simulink model "Drone2_simulink_old1"  (R2024b)
settings: Solver=ode1be  StartTime=0.0  StopTime=1200  FixedStep=0.001  MaxStep=0.001  MinStep=0.00095  RelTol=1e-3
undefined symbols (not defined in the file): DiscIntNeverNeededParam, Environment, Newton, Raphson, Sim3dSensor, Vehicle, X, Y, Z
libraries: sm_lib x2951, nesl_utility x76, slpidlib x25, simulink x4, eeGeneralControl x4, matrix_library x3, rllib x2, sim3dlib x2, uavsim3dlib x2, dspstat3 x1, SignalEditorBlockLib x1, sharedutil x1
(part 9 of 21)

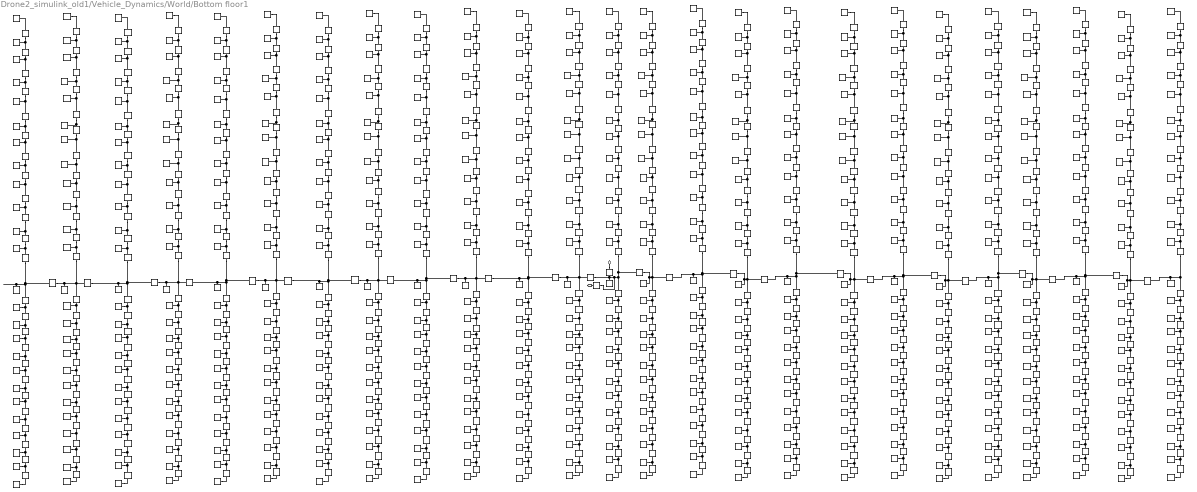
== system Drone2_simulink_old1/Vehicle_Dynamics/World/Bottom floor1 ==
  Brick Solid : sm_lib/Body Elements/Brick Solid  BrickDimensions=[25*X 25*Y Z]  BrickDimensionsUnits=m  ExportEntireGeometry=on  InertiaType=CalculateFromGeometry  BasedOnType=Density  Density=10000  DensityUnits=kg/m^3  Mass=1  MassUnits=kg  CenterOfMass=[0 0 0]  CenterOfMassUnits=m  MomentsOfInertia=[1 1 1]  MomentsOfInertiaUnits=kg*m^2  ProductsOfInertia=[0 0 0]  ProductsOfInertiaUnits=kg*m^2  GraphicType=FromGeometry  MarkerShape=Sphere  MarkerSize=10  GraphicVisPropType=SimpleVisualProperties  GraphicDiffuseColor=[1.0 1.0 1.0]  GraphicOpacity=0  GraphicSpecularColor=[0.5 0.5 0.5 1.0]  GraphicAmbientColor=[0.15 0.15 0.15 1.0]  GraphicEmissiveColor=[0.0 0.0 0.0 1.0]  GraphicShininess=75  DoExposeReferenceFrame=on  SerializedFrames=<Frames/>
  Rigid Transform : sm_lib/Frames and Transforms/Rigid Transform  RotationMethod=None  FollAlignAxisA=+X  BaseAlignAxisA=+Y  FollAlignAxisB=+Y  BaseAlignAxisB=+Z  RotationStandardAxis=+Z  RotationAngle=0  RotationAngleUnits=deg  RotationArbitraryAxis=[0 0 1]  RotationSequenceAxes=FollowerAxes  RotationSequence=XYX  RotationSequenceAngles=[0 0 0]  RotationSequenceAnglesUnits=deg  RotationMatrix=[1 0 0;0 1 0;0 0 1]  Quaternion=[1 0 0 0]  TranslationMethod=Cartesian  TranslationCartesianOffset=[0 0 ZB]  TranslationCartesianOffsetUnits=m  TranslationStandardAxis=+Z  TranslationStandardOffset=0  TranslationStandardOffsetUnits=m  TranslationROffset=0  TranslationROffsetUnits=m  TranslationThetaOffset=0  TranslationThetaOffsetUnits=deg  TranslationZOffset=0  TranslationZOffsetUnits=m
  Rigid Transform{1,5,7,9..10,12..13,15..16,18..19,21} (12 alike) : sm_lib/Frames and Transforms/Rigid Transform  RotationMethod=None  FollAlignAxisA=+X  BaseAlignAxisA=+Y  FollAlignAxisB=+Y  BaseAlignAxisB=+Z  RotationStandardAxis=+Z  RotationAngle=0  RotationAngleUnits=deg  RotationArbitraryAxis=[0 0 1]  RotationSequenceAxes=FollowerAxes  RotationSequence=XYX  RotationSequenceAngles=[0 0 0]  RotationSequenceAnglesUnits=deg  RotationMatrix=[1 0 0;0 1 0;0 0 1]  Quaternion=[1 0 0 0]  TranslationMethod=Cartesian  TranslationCartesianOffset=[X 0 0]  TranslationCartesianOffsetUnits=m  TranslationStandardAxis=+Z  TranslationStandardOffset=0  TranslationStandardOffsetUnits=m  TranslationROffset=0  TranslationROffsetUnits=m  TranslationThetaOffset=0  TranslationThetaOffsetUnits=deg  TranslationZOffset=0  TranslationZOffsetUnits=m
  Rigid Transform{2..4,6,8,11,14,17,20,22..24} (12 alike) : sm_lib/Frames and Transforms/Rigid Transform  RotationMethod=None  FollAlignAxisA=+X  BaseAlignAxisA=+Y  FollAlignAxisB=+Y  BaseAlignAxisB=+Z  RotationStandardAxis=+Z  RotationAngle=0  RotationAngleUnits=deg  RotationArbitraryAxis=[0 0 1]  RotationSequenceAxes=FollowerAxes  RotationSequence=XYX  RotationSequenceAngles=[0 0 0]  RotationSequenceAnglesUnits=deg  RotationMatrix=[1 0 0;0 1 0;0 0 1]  Quaternion=[1 0 0 0]  TranslationMethod=Cartesian  TranslationCartesianOffset=[-X 0 0]  TranslationCartesianOffsetUnits=m  TranslationStandardAxis=+Z  TranslationStandardOffset=0  TranslationStandardOffsetUnits=m  TranslationROffset=0  TranslationROffsetUnits=m  TranslationThetaOffset=0  TranslationThetaOffsetUnits=deg  TranslationZOffset=0  TranslationZOffsetUnits=m
  bottom{,3..4,6,8,10,13,15,17,19,21,23..25,27,30,32,34,36,41..44,46,48,50,52,55,57,59,61,66..69,71,73,75,77,80,82,84,86,89,91..94,96,98,100,102,105,107,109,111,114,116..119,121,123,125,127,130,132,134,136,141..144,146,148,150,152,155,157,159,161,164,166..169,171,173,175,177,180,182,184,186,191..194,196,198,200,202,205,207,209,211,214,216..219,221,223,225,227,230,232,234,236,241..244,246,248,250,252,255,257,259,261,264,266..269,271,273,275,277,280,282,284,286,291..294,296,298,300,302,305,307,309,311,314,316..319,321,323,325,327,330,332,334,336,341..344,346,348,350,352,355,357,359,361,364,366..369,371,373,375,377,380,382,384,386,389,391..394,396,398,400,402,405,407,409,411,416..419,421,423,425,427,430,432,434,436,439,441..444,446,448,450,452,455,457,459,461,464,466..469,471,473,475,477,480,482,484,486,491..494,496,498,500,502,505,507,509,511,516..519,521,523,525,527,530,532,534,536,539,541..544,546,548,550,552,555,557,559,561,564,566..569,571,573,575,577,580,582,584,586,591..594,596,598,600,602,605,607,609,611,616..619,621,623} (313 alike) : sm_lib/Body Elements/Brick Solid  BrickDimensions=[X Y Z]  BrickDimensionsUnits=m  ExportEntireGeometry=off  InertiaType=CalculateFromGeometry  BasedOnType=Density  Density=1  DensityUnits=kg/m^3  Mass=1  MassUnits=kg  CenterOfMass=[0 0 0]  CenterOfMassUnits=m  MomentsOfInertia=[1 1 1]  MomentsOfInertiaUnits=kg*m^2  ProductsOfInertia=[0 0 0]  ProductsOfInertiaUnits=kg*m^2  GraphicType=FromGeometry  MarkerShape=Sphere  MarkerSize=10  GraphicVisPropType=SimpleVisualProperties  GraphicDiffuseColor=Color1  GraphicOpacity=1  GraphicSpecularColor=[0.5 0.5 0.5 1.0]  GraphicAmbientColor=[0.15 0.15 0.15 1.0]  GraphicEmissiveColor=[0.0 0.0 0.0 1.0]  GraphicShininess=75  DoExposeReferenceFrame=on  SerializedFrames=<Frames/>
  bottom{1..2,5,7,9,11..12,14,16,18,20,22,26,28..29,31,33,35,37..40,45,47,49,51,53..54,56,58,60,62..65,70,72,74,76,78..79,81,83,85,87..88,90,95,97,99,101,103..104,106,108,110,112..113,115,120,122,124,126,128..129,131,133,135,137..140,145,147,149,151,153..154,156,158,160,162..163,165,170,172,174,176,178..179,181,183,185,187..190,195,197,199,201,203..204,206,208,210,212..213,215,220,222,224,226,228..229,231,233,235,237..240,245,247,249,251,253..254,256,258,260,262..263,265,270,272,274,276,278..279,281,283,285,287..290,295,297,299,301,303..304,306,308,310,312..313,315,320,322,324,326,328..329,331,333,335,337..340,345,347,349,351,353..354,356,358,360,362..363,365,370,372,374,376,378..379,381,383,385,387..388,390,395,397,399,401,403..404,406,408,410,412..415,420,422,424,426,428..429,431,433,435,437..438,440,445,447,449,451,453..454,456,458,460,462..463,465,470,472,474,476,478..479,481,483,485,487..490,495,497,499,501,503..504,506,508,510,512..515,520,522,524,526,528..529,531,533,535,537..538,540,545,547,549,551,553..554,556,558,560,562..563,565,570,572,574,576,578..579,581,583,585,587..590,595,597,599,601,603..604,606,608,610,612..615,620,622,624} (312 alike) : sm_lib/Body Elements/Brick Solid  BrickDimensions=[X Y Z]  BrickDimensionsUnits=m  ExportEntireGeometry=off  InertiaType=CalculateFromGeometry  BasedOnType=Density  Density=1  DensityUnits=kg/m^3  Mass=1  MassUnits=kg  CenterOfMass=[0 0 0]  CenterOfMassUnits=m  MomentsOfInertia=[1 1 1]  MomentsOfInertiaUnits=kg*m^2  ProductsOfInertia=[0 0 0]  ProductsOfInertiaUnits=kg*m^2  GraphicType=FromGeometry  MarkerShape=Sphere  MarkerSize=10  GraphicVisPropType=SimpleVisualProperties  GraphicDiffuseColor=Color2  GraphicOpacity=1  GraphicSpecularColor=[0.5 0.5 0.5 1.0]  GraphicAmbientColor=[0.15 0.15 0.15 1.0]  GraphicEmissiveColor=[0.0 0.0 0.0 1.0]  GraphicShininess=75  DoExposeReferenceFrame=on  SerializedFrames=<Frames/>
  water surface ti bottom{1..2,4..5,7..10,12..13,18,24,26,28..29,34,36..37,41,43..44,46..48,50,52..53,58,60..61,65,67..68,70..74,76..77,82,84,89,91..92,94..98,100..101,106,108,113,115..116,118..120,122,124..125,130,132..133,137,139..140,142..146,148..149,154,156,161,163..164,166..168,170,172..173,178,180..181,185,187..188,190..194,196..197,202,204,209,211..212,214..216,218,220..221,226,228..229,233,235..236,238..242,244..245,250,252,257,259..260,262..264,266,268..269,274,276..277,281,283..284,286..290,292..293,298,300,305,307..308,310..312,314,316..317,322,324..325,329,331..332,334..338,340..341,346,348,353,355..356,358..362,367,369,374,376..377,379..381,383,385..386,391,393..394,398,400..401,403..407,409..410,415,417,422,424..425,427..431,436,438,443,445..446,448..450,452,454..455,460,462..463,467,469..470,472..476,479,481..482,487,489..490,494,496..497,499..503,505..506,511,513,518,520..521,523..527,532,534,539,541..542,544..546,548,550..551,556,558..559,563,565..566,568..572,575,577..578,583,585..586,590,592..593,595..599} (300 alike) : sm_lib/Frames and Transforms/Rigid Transform  RotationMethod=None  FollAlignAxisA=+X  BaseAlignAxisA=+Y  FollAlignAxisB=+Y  BaseAlignAxisB=+Z  RotationStandardAxis=+Z  RotationAngle=0  RotationAngleUnits=deg  RotationArbitraryAxis=[0 0 1]  RotationSequenceAxes=FollowerAxes  RotationSequence=XYX  RotationSequenceAngles=[0 0 0]  RotationSequenceAnglesUnits=deg  RotationMatrix=[1 0 0;0 1 0;0 0 1]  Quaternion=[1 0 0 0]  TranslationMethod=Cartesian  TranslationCartesianOffset=[0 Y 0]  TranslationCartesianOffsetUnits=m  TranslationStandardAxis=+Z  TranslationStandardOffset=0  TranslationStandardOffsetUnits=m  TranslationROffset=0  TranslationROffsetUnits=m  TranslationThetaOffset=0  TranslationThetaOffsetUnits=deg  TranslationZOffset=0  TranslationZOffsetUnits=m
  water surface ti bottom{3,6,11,14..17,19..23,25,27,30..33,35,38..40,42,45,49,51,54..57,59,62..64,66,69,75,78..81,83,85..88,90,93,99,102..105,107,109..112,114,117,121,123,126..129,131,134..136,138,141,147,150..153,155,157..160,162,165,169,171,174..177,179,182..184,186,189,195,198..201,203,205..208,210,213,217,219,222..225,227,230..232,234,237,243,246..249,251,253..256,258,261,265,267,270..273,275,278..280,282,285,291,294..297,299,301..304,306,309,313,315,318..321,323,326..328,330,333,339,342..345,347,349..352,354,357,363..366,368,370..373,375,378,382,384,387..390,392,395..397,399,402,408,411..414,416,418..421,423,426,432..435,437,439..442,444,447,451,453,456..459,461,464..466,468,471,477..478,480,483..486,488,491..493,495,498,504,507..510,512,514..517,519,522,528..531,533,535..538,540,543,547,549,552..555,557,560..562,564,567,573..574,576,579..582,584,587..589,591,594,600} (300 alike) : sm_lib/Frames and Transforms/Rigid Transform  RotationMethod=None  FollAlignAxisA=+X  BaseAlignAxisA=+Y  FollAlignAxisB=+Y  BaseAlignAxisB=+Z  RotationStandardAxis=+Z  RotationAngle=0  RotationAngleUnits=deg  RotationArbitraryAxis=[0 0 1]  RotationSequenceAxes=FollowerAxes  RotationSequence=XYX  RotationSequenceAngles=[0 0 0]  RotationSequenceAnglesUnits=deg  RotationMatrix=[1 0 0;0 1 0;0 0 1]  Quaternion=[1 0 0 0]  TranslationMethod=Cartesian  TranslationCartesianOffset=[0 -Y 0]  TranslationCartesianOffsetUnits=m  TranslationStandardAxis=+Z  TranslationStandardOffset=0  TranslationStandardOffsetUnits=m  TranslationROffset=0  TranslationROffsetUnits=m  TranslationThetaOffset=0  TranslationThetaOffsetUnits=deg  TranslationZOffset=0  TranslationZOffsetUnits=m
  From World : PMIOPort  Side=Left
  Collision : PMIOPort  Port=2  Side=Right
  connections:
  Collision/RConn1 -- Brick Solid/LConn1
  bottom539/RConn1 -- water surface ti bottom514/RConn1
  water surface ti bottom539/RConn1 -- bottom567/RConn1
  water surface ti bottom518/RConn1 -- bottom542/RConn1
  bottom589/RConn1 -- water surface ti bottom559/RConn1
  bottom588/RConn1 -- water surface ti bottom560/RConn1
  bottom564/RConn1 -- water surface ti bottom535/RConn1
  bottom613/RConn1 -- water surface ti bottom587/RConn1
  bottom614/RConn1 -- water surface ti bottom586/RConn1
  water surface ti bottom535/LConn1 -- water surface ti bottom536/RConn1 -- bottom563/RConn1
  water surface ti bottom536/LConn1 -- bottom566/RConn1 -- water surface ti bottom537/RConn1
  water surface ti bottom537/LConn1 -- bottom565/RConn1 -- water surface ti bottom538/RConn1
  water surface ti bottom529/RConn1 -- bottom559/RConn1 -- water surface ti bottom538/LConn1
  water surface ti bottom529/LConn1 -- bottom558/RConn1 -- water surface ti bottom530/RConn1
  water surface ti bottom530/LConn1 -- water surface ti bottom531/RConn1 -- bottom561/RConn1
  water surface ti bottom531/LConn1 -- water surface ti bottom533/RConn1 -- bottom560/RConn1
  water surface ti bottom533/LConn1 -- bottom557/RConn1 -- water surface ti bottom573/RConn1
  water surface ti bottom573/LConn1 -- water surface ti bottom528/RConn1 -- bottom554/RConn1
  water surface ti bottom539/LConn1 -- bottom556/RConn1 -- water surface ti bottom527/RConn1
  water surface ti bottom527/LConn1 -- water surface ti bottom526/RConn1 -- bottom555/RConn1
  bottom553/RConn1 -- water surface ti bottom526/LConn1 -- water surface ti bottom532/RConn1
  water surface ti bottom532/LConn1 -- bottom552/RConn1 -- water surface ti bottom572/RConn1
  water surface ti bottom546/RConn1 -- bottom574/RConn1 -- water surface ti bottom572/LConn1
  water surface ti bottom545/RConn1 -- bottom573/RConn1 -- water surface ti bottom546/LConn1
  water surface ti bottom545/LConn1 -- water surface ti bottom544/RConn1 -- bottom572/RConn1
  water surface ti bottom542/RConn1 -- bottom571/RConn1 -- water surface ti bottom544/LConn1
  water surface ti bottom542/LConn1 -- water surface ti bottom541/RConn1 -- bottom570/RConn1
  water surface ti bottom528/LConn1 -- bottom569/RConn1 -- water surface ti bottom540/RConn1
  water surface ti bottom534/RConn1 -- bottom568/RConn1 -- water surface ti bottom541/LConn1
  bottom550/RConn1 -- water surface ti bottom543/LConn1 -- water surface ti bottom571/LConn1 -- Rigid Transform23/RConn1
  water surface ti bottom571/RConn1 -- bottom551/RConn1 -- water surface ti bottom534/LConn1
  water surface ti bottom540/LConn1 -- bottom562/RConn1 -- water surface ti bottom543/RConn1
  water surface ti bottom559/LConn1 -- water surface ti bottom563/RConn1 -- bottom592/RConn1
  water surface ti bottom560/LConn1 -- bottom591/RConn1 -- water surface ti bottom561/RConn1
  water surface ti bottom561/LConn1 -- bottom590/RConn1 -- water surface ti bottom562/RConn1
  water surface ti bottom553/RConn1 -- bottom584/RConn1 -- water surface ti bottom562/LConn1
  water surface ti bottom553/LConn1 -- bottom583/RConn1 -- water surface ti bottom554/RConn1
  water surface ti bottom554/LConn1 -- water surface ti bottom555/RConn1 -- bottom586/RConn1
  water surface ti bottom555/LConn1 -- water surface ti bottom557/RConn1 -- bottom585/RConn1
  water surface ti bottom557/LConn1 -- bottom582/RConn1 -- water surface ti bottom549/RConn1
  water surface ti bottom549/LConn1 -- water surface ti bottom552/RConn1 -- bottom579/RConn1
  water surface ti bottom551/RConn1 -- water surface ti bottom563/LConn1 -- bottom581/RConn1
  water surface ti bottom550/RConn1 -- water surface ti bottom551/LConn1 -- bottom580/RConn1
  water surface ti bottom556/RConn1 -- water surface ti bottom550/LConn1 -- bottom578/RConn1
  water surface ti bottom548/RConn1 -- water surface ti bottom556/LConn1 -- bottom577/RConn1
  water surface ti bottom548/LConn1 -- water surface ti bottom570/RConn1 -- bottom599/RConn1
  water surface ti bottom570/LConn1 -- water surface ti bottom569/RConn1 -- bottom598/RConn1
  water surface ti bottom568/RConn1 -- water surface ti bottom569/LConn1 -- bottom597/RConn1
  water surface ti bottom566/RConn1 -- water surface ti bottom568/LConn1 -- bottom596/RConn1
  water surface ti bottom565/RConn1 -- water surface ti bottom566/LConn1 -- bottom595/RConn1
  water surface ti bottom552/LConn1 -- bottom594/RConn1 -- water surface ti bottom564/RConn1
  water surface ti bottom558/RConn1 -- water surface ti bottom565/LConn1 -- bottom593/RConn1
  water surface ti bottom567/LConn1 -- water surface ti bottom547/RConn1 -- bottom575/RConn1
  Rigid Transform20/RConn1 -- water surface ti bottom558/LConn1 -- Rigid Transform23/LConn1 -- bottom576/RConn1 -- water surface ti bottom547/LConn1
  bottom587/RConn1 -- water surface ti bottom564/LConn1 -- water surface ti bottom567/RConn1
  water surface ti bottom514/LConn1 -- bottom538/RConn1 -- water surface ti bottom515/RConn1
  water surface ti bottom515/LConn1 -- water surface ti bottom516/RConn1 -- bottom541/RConn1
  water surface ti bottom516/LConn1 -- water surface ti bottom517/RConn1 -- bottom540/RConn1
  water surface ti bottom508/RConn1 -- water surface ti bottom517/LConn1 -- bottom534/RConn1
  water surface ti bottom508/LConn1 -- water surface ti bottom509/RConn1 -- bottom533/RConn1
  water surface ti bottom509/LConn1 -- bottom536/RConn1 -- water surface ti bottom510/RConn1
  water surface ti bottom510/LConn1 -- bottom535/RConn1 -- water surface ti bottom512/RConn1
  water surface ti bottom512/LConn1 -- water surface ti bottom600/RConn1 -- bottom532/RConn1
  water surface ti bottom600/LConn1 -- bottom529/RConn1 -- water surface ti bottom507/RConn1
  water surface ti bottom518/LConn1 -- water surface ti bottom506/RConn1 -- bottom531/RConn1
  water surface ti bottom506/LConn1 -- bottom530/RConn1 -- water surface ti bottom505/RConn1
  bottom528/RConn1 -- water surface ti bottom511/RConn1 -- water surface ti bottom505/LConn1
  water surface ti bottom511/LConn1 -- water surface ti bottom599/RConn1 -- bottom527/RConn1
  water surface ti bottom525/RConn1 -- water surface ti bottom599/LConn1 -- bottom549/RConn1
  water surface ti bottom524/RConn1 -- water surface ti bottom525/LConn1 -- bottom548/RConn1
  water surface ti bottom524/LConn1 -- bottom547/RConn1 -- water surface ti bottom523/RConn1
  water surface ti bottom521/RConn1 -- water surface ti bottom523/LConn1 -- bottom546/RConn1
  water surface ti bottom521/LConn1 -- bottom545/RConn1 -- water surface ti bottom520/RConn1
  water surface ti bottom507/LConn1 -- water surface ti bottom519/RConn1 -- bottom544/RConn1
  water surface ti bottom513/RConn1 -- water surface ti bottom520/LConn1 -- bottom543/RConn1
  water surface ti bottom598/LConn1 -- water surface ti bottom522/LConn1 -- bottom525/RConn1 -- Rigid Transform20/LConn1 -- Rigid Transform14/RConn1
  water surface ti bottom598/RConn1 -- water surface ti bottom513/LConn1 -- bottom526/RConn1
  water surface ti bottom519/LConn1 -- water surface ti bottom522/RConn1 -- bottom537/RConn1
  water surface ti bottom586/LConn1 -- bottom617/RConn1 -- water surface ti bottom590/RConn1
  water surface ti bottom587/LConn1 -- water surface ti bottom588/RConn1 -- bottom616/RConn1
  water surface ti bottom588/LConn1 -- water surface ti bottom589/RConn1 -- bottom615/RConn1
  water surface ti bottom580/RConn1 -- water surface ti bottom589/LConn1 -- bottom609/RConn1
  water surface ti bottom580/LConn1 -- water surface ti bottom581/RConn1 -- bottom608/RConn1
  water surface ti bottom581/LConn1 -- bottom611/RConn1 -- water surface ti bottom582/RConn1
  water surface ti bottom582/LConn1 -- bottom610/RConn1 -- water surface ti bottom584/RConn1
  water surface ti bottom584/LConn1 -- water surface ti bottom576/RConn1 -- bottom607/RConn1
  water surface ti bottom576/LConn1 -- bottom604/RConn1 -- water surface ti bottom579/RConn1
  water surface ti bottom578/RConn1 -- bottom606/RConn1 -- water surface ti bottom590/LConn1
  water surface ti bottom577/RConn1 -- bottom605/RConn1 -- water surface ti bottom578/LConn1
  water surface ti bottom583/RConn1 -- bottom603/RConn1 -- water surface ti bottom577/LConn1
  water surface ti bottom575/RConn1 -- bottom602/RConn1 -- water surface ti bottom583/LConn1
  water surface ti bottom575/LConn1 -- bottom624/RConn1 -- water surface ti bottom597/RConn1
  water surface ti bottom597/LConn1 -- bottom623/RConn1 -- water surface ti bottom596/RConn1
  water surface ti bottom595/RConn1 -- bottom622/RConn1 -- water surface ti bottom596/LConn1
  water surface ti bottom593/RConn1 -- bottom621/RConn1 -- water surface ti bottom595/LConn1
  water surface ti bottom592/RConn1 -- bottom620/RConn1 -- water surface ti bottom593/LConn1
  water surface ti bottom579/LConn1 -- water surface ti bottom591/RConn1 -- bottom619/RConn1
  water surface ti bottom585/RConn1 -- bottom618/RConn1 -- water surface ti bottom592/LConn1
  water surface ti bottom594/LConn1 -- bottom600/RConn1 -- water surface ti bottom574/RConn1
  Rigid Transform14/LConn1 -- water surface ti bottom585/LConn1 -- Rigid Transform17/RConn1 -- water surface ti bottom574/LConn1 -- bottom601/RConn1
  bottom612/RConn1 -- water surface ti bottom594/RConn1 -- water surface ti bottom591/LConn1
  bottom514/RConn1 -- water surface ti bottom490/RConn1
  bottom513/RConn1 -- water surface ti bottom491/RConn1
  water surface ti bottom422/RConn1 -- bottom442/RConn1
  bottom439/RConn1 -- water surface ti bottom418/RConn1
  bottom464/RConn1 -- water surface ti bottom439/RConn1
  water surface ti bottom443/RConn1 -- bottom467/RConn1
  bottom488/RConn1 -- water surface ti bottom464/RConn1
  bottom489/RConn1 -- water surface ti bottom463/RConn1
  water surface ti bottom439/LConn1 -- bottom463/RConn1 -- water surface ti bottom440/RConn1
  water surface ti bottom440/LConn1 -- water surface ti bottom441/RConn1 -- bottom466/RConn1
  water surface ti bottom441/LConn1 -- water surface ti bottom442/RConn1 -- bottom465/RConn1
  water surface ti bottom433/RConn1 -- water surface ti bottom442/LConn1 -- bottom459/RConn1
  water surface ti bottom433/LConn1 -- water surface ti bottom434/RConn1 -- bottom458/RConn1
  water surface ti bottom434/LConn1 -- bottom461/RConn1 -- water surface ti bottom435/RConn1
  water surface ti bottom435/LConn1 -- bottom460/RConn1 -- water surface ti bottom437/RConn1
  water surface ti bottom437/LConn1 -- water surface ti bottom477/RConn1 -- bottom457/RConn1
  water surface ti bottom477/LConn1 -- bottom454/RConn1 -- water surface ti bottom432/RConn1
  water surface ti bottom443/LConn1 -- water surface ti bottom431/RConn1 -- bottom456/RConn1
  water surface ti bottom431/LConn1 -- bottom455/RConn1 -- water surface ti bottom430/RConn1
  bottom453/RConn1 -- water surface ti bottom436/RConn1 -- water surface ti bottom430/LConn1
  water surface ti bottom436/LConn1 -- water surface ti bottom476/RConn1 -- bottom452/RConn1
  water surface ti bottom450/RConn1 -- water surface ti bottom476/LConn1 -- bottom474/RConn1
  water surface ti bottom449/RConn1 -- water surface ti bottom450/LConn1 -- bottom473/RConn1
  water surface ti bottom449/LConn1 -- bottom472/RConn1 -- water surface ti bottom448/RConn1
  water surface ti bottom446/RConn1 -- water surface ti bottom448/LConn1 -- bottom471/RConn1
  water surface ti bottom446/LConn1 -- bottom470/RConn1 -- water surface ti bottom445/RConn1
  water surface ti bottom432/LConn1 -- water surface ti bottom444/RConn1 -- bottom469/RConn1
  water surface ti bottom438/RConn1 -- water surface ti bottom445/LConn1 -- bottom468/RConn1
  water surface ti bottom475/LConn1 -- water surface ti bottom447/LConn1 -- bottom450/RConn1 -- Rigid Transform17/LConn1 -- Rigid Transform8/RConn1
  water surface ti bottom475/RConn1 -- water surface ti bottom438/LConn1 -- bottom451/RConn1
  water surface ti bottom444/LConn1 -- water surface ti bottom447/RConn1 -- bottom462/RConn1
  water surface ti bottom463/LConn1 -- bottom492/RConn1 -- water surface ti bottom467/RConn1
  water surface ti bottom464/LConn1 -- water surface ti bottom465/RConn1 -- bottom491/RConn1
  water surface ti bottom465/LConn1 -- water surface ti bottom466/RConn1 -- bottom490/RConn1
  water surface ti bottom457/RConn1 -- water surface ti bottom466/LConn1 -- bottom484/RConn1
  water surface ti bottom457/LConn1 -- water surface ti bottom458/RConn1 -- bottom483/RConn1
  water surface ti bottom458/LConn1 -- bottom486/RConn1 -- water surface ti bottom459/RConn1
  water surface ti bottom459/LConn1 -- bottom485/RConn1 -- water surface ti bottom461/RConn1
  water surface ti bottom461/LConn1 -- water surface ti bottom453/RConn1 -- bottom482/RConn1
  water surface ti bottom453/LConn1 -- bottom479/RConn1 -- water surface ti bottom456/RConn1
  water surface ti bottom455/RConn1 -- bottom481/RConn1 -- water surface ti bottom467/LConn1
  water surface ti bottom454/RConn1 -- bottom480/RConn1 -- water surface ti bottom455/LConn1
  water surface ti bottom460/RConn1 -- bottom478/RConn1 -- water surface ti bottom454/LConn1
  water surface ti bottom452/RConn1 -- bottom477/RConn1 -- water surface ti bottom460/LConn1
  water surface ti bottom452/LConn1 -- bottom499/RConn1 -- water surface ti bottom474/RConn1
  water surface ti bottom474/LConn1 -- bottom498/RConn1 -- water surface ti bottom473/RConn1
  water surface ti bottom472/RConn1 -- bottom497/RConn1 -- water surface ti bottom473/LConn1
  water surface ti bottom470/RConn1 -- bottom496/RConn1 -- water surface ti bottom472/LConn1
  water surface ti bottom469/RConn1 -- bottom495/RConn1 -- water surface ti bottom470/LConn1
  water surface ti bottom456/LConn1 -- water surface ti bottom468/RConn1 -- bottom494/RConn1
  water surface ti bottom462/RConn1 -- bottom493/RConn1 -- water surface ti bottom469/LConn1
  water surface ti bottom471/LConn1 -- bottom475/RConn1 -- water surface ti bottom451/RConn1
  Rigid Transform8/LConn1 -- water surface ti bottom462/LConn1 -- Rigid Transform4/RConn1 -- water surface ti bottom451/LConn1 -- bottom476/RConn1
  bottom487/RConn1 -- water surface ti bottom471/RConn1 -- water surface ti bottom468/LConn1
  water surface ti bottom418/LConn1 -- water surface ti bottom419/RConn1 -- bottom438/RConn1
  water surface ti bottom419/LConn1 -- bottom441/RConn1 -- water surface ti bottom420/RConn1
  water surface ti bottom420/LConn1 -- bottom440/RConn1 -- water surface ti bottom421/RConn1
  water surface ti bottom412/RConn1 -- bottom434/RConn1 -- water surface ti bottom421/LConn1
  water surface ti bottom412/LConn1 -- bottom433/RConn1 -- water surface ti bottom413/RConn1
  water surface ti bottom413/LConn1 -- water surface ti bottom414/RConn1 -- bottom436/RConn1
  water surface ti bottom414/LConn1 -- water surface ti bottom416/RConn1 -- bottom435/RConn1
  water surface ti bottom416/LConn1 -- bottom432/RConn1 -- water surface ti bottom504/RConn1
  water surface ti bottom504/LConn1 -- water surface ti bottom411/RConn1 -- bottom429/RConn1
  water surface ti bottom422/LConn1 -- bottom431/RConn1 -- water surface ti bottom410/RConn1
  water surface ti bottom410/LConn1 -- water surface ti bottom409/RConn1 -- bottom430/RConn1
  bottom428/RConn1 -- water surface ti bottom409/LConn1 -- water surface ti bottom415/RConn1
  water surface ti bottom415/LConn1 -- bottom427/RConn1 -- water surface ti bottom503/RConn1
  water surface ti bottom429/RConn1 -- bottom449/RConn1 -- water surface ti bottom503/LConn1
  water surface ti bottom428/RConn1 -- bottom448/RConn1 -- water surface ti bottom429/LConn1
  water surface ti bottom428/LConn1 -- water surface ti bottom427/RConn1 -- bottom447/RConn1
  water surface ti bottom425/RConn1 -- bottom446/RConn1 -- water surface ti bottom427/LConn1
  water surface ti bottom425/LConn1 -- water surface ti bottom424/RConn1 -- bottom445/RConn1
  water surface ti bottom411/LConn1 -- bottom444/RConn1 -- water surface ti bottom423/RConn1
  water surface ti bottom417/RConn1 -- bottom443/RConn1 -- water surface ti bottom424/LConn1
  bottom425/RConn1 -- water surface ti bottom426/LConn1 -- water surface ti bottom502/LConn1 -- Rigid Transform11/RConn1 -- Rigid Transform4/LConn1
  water surface ti bottom502/RConn1 -- bottom426/RConn1 -- water surface ti bottom417/LConn1
  water surface ti bottom423/LConn1 -- bottom437/RConn1 -- water surface ti bottom426/RConn1
  water surface ti bottom490/LConn1 -- water surface ti bottom494/RConn1 -- bottom517/RConn1
  water surface ti bottom491/LConn1 -- bottom516/RConn1 -- water surface ti bottom492/RConn1
  water surface ti bottom492/LConn1 -- bottom515/RConn1 -- water surface ti bottom493/RConn1
  water surface ti bottom484/RConn1 -- bottom509/RConn1 -- water surface ti bottom493/LConn1
  water surface ti bottom484/LConn1 -- bottom508/RConn1 -- water surface ti bottom485/RConn1
  water surface ti bottom485/LConn1 -- water surface ti bottom486/RConn1 -- bottom511/RConn1
  water surface ti bottom486/LConn1 -- water surface ti bottom488/RConn1 -- bottom510/RConn1
  water surface ti bottom488/LConn1 -- bottom507/RConn1 -- water surface ti bottom480/RConn1
  water surface ti bottom480/LConn1 -- water surface ti bottom483/RConn1 -- bottom504/RConn1
  water surface ti bottom482/RConn1 -- water surface ti bottom494/LConn1 -- bottom506/RConn1
  water surface ti bottom481/RConn1 -- water surface ti bottom482/LConn1 -- bottom505/RConn1
  water surface ti bottom487/RConn1 -- water surface ti bottom481/LConn1 -- bottom503/RConn1
  water surface ti bottom479/RConn1 -- water surface ti bottom487/LConn1 -- bottom502/RConn1
  water surface ti bottom479/LConn1 -- water surface ti bottom501/RConn1 -- bottom524/RConn1
  water surface ti bottom501/LConn1 -- water surface ti bottom500/RConn1 -- bottom523/RConn1
  water surface ti bottom499/RConn1 -- water surface ti bottom500/LConn1 -- bottom522/RConn1
  water surface ti bottom497/RConn1 -- water surface ti bottom499/LConn1 -- bottom521/RConn1
  water surface ti bottom496/RConn1 -- water surface ti bottom497/LConn1 -- bottom520/RConn1
  water surface ti bottom483/LConn1 -- bottom519/RConn1 -- water surface ti bottom495/RConn1
  water surface ti bottom489/RConn1 -- water surface ti bottom496/LConn1 -- bottom518/RConn1
  water surface ti bottom498/LConn1 -- water surface ti bottom478/RConn1 -- bottom500/RConn1
  Rigid Transform11/LConn1 -- bottom501/RConn1 -- Rigid Transform3/RConn1 -- water surface ti bottom489/LConn1 -- water surface ti bottom478/LConn1
  bottom512/RConn1 -- water surface ti bottom495/LConn1 -- water surface ti bottom498/RConn1
  bottom414/RConn1 -- water surface ti bottom394/RConn1
  bottom413/RConn1 -- water surface ti bottom395/RConn1
  water surface ti bottom374/RConn1 -- bottom392/RConn1
  bottom389/RConn1 -- water surface ti bottom370/RConn1
  water surface ti bottom370/LConn1 -- water surface ti bottom371/RConn1 -- bottom388/RConn1
  water surface ti bottom371/LConn1 -- bottom391/RConn1 -- water surface ti bottom372/RConn1
  water surface ti bottom372/LConn1 -- bottom390/RConn1 -- water surface ti bottom373/RConn1
  water surface ti bottom364/RConn1 -- bottom384/RConn1 -- water surface ti bottom373/LConn1
  water surface ti bottom364/LConn1 -- bottom383/RConn1 -- water surface ti bottom365/RConn1
  water surface ti bottom365/LConn1 -- water surface ti bottom366/RConn1 -- bottom386/RConn1
  water surface ti bottom366/LConn1 -- water surface ti bottom368/RConn1 -- bottom385/RConn1
  water surface ti bottom368/LConn1 -- bottom382/RConn1 -- water surface ti bottom408/RConn1
  water surface ti bottom408/LConn1 -- water surface ti bottom363/RConn1 -- bottom379/RConn1
  water surface ti bottom374/LConn1 -- bottom381/RConn1 -- water surface ti bottom362/RConn1
  water surface ti bottom362/LConn1 -- water surface ti bottom361/RConn1 -- bottom380/RConn1
  bottom378/RConn1 -- water surface ti bottom361/LConn1 -- water surface ti bottom367/RConn1
  water surface ti bottom367/LConn1 -- bottom377/RConn1 -- water surface ti bottom407/RConn1
  water surface ti bottom381/RConn1 -- bottom399/RConn1 -- water surface ti bottom407/LConn1
  water surface ti bottom380/RConn1 -- bottom398/RConn1 -- water surface ti bottom381/LConn1
  water surface ti bottom380/LConn1 -- water surface ti bottom379/RConn1 -- bottom397/RConn1
  water surface ti bottom377/RConn1 -- bottom396/RConn1 -- water surface ti bottom379/LConn1
  water surface ti bottom377/LConn1 -- water surface ti bottom376/RConn1 -- bottom395/RConn1
  water surface ti bottom363/LConn1 -- bottom394/RConn1 -- water surface ti bottom375/RConn1
  water surface ti bottom369/RConn1 -- bottom393/RConn1 -- water surface ti bottom376/LConn1
  water surface ti bottom378/LConn1 -- water surface ti bottom406/LConn1 -- Rigid Transform24/RConn1 -- Rigid Transform3/LConn1 -- bottom375/RConn1
  water surface ti bottom406/RConn1 -- bottom376/RConn1 -- water surface ti bottom369/LConn1
  water surface ti bottom375/LConn1 -- bottom387/RConn1 -- water surface ti bottom378/RConn1
  water surface ti bottom394/LConn1 -- water surface ti bottom398/RConn1 -- bottom417/RConn1
  water surface ti bottom395/LConn1 -- bottom416/RConn1 -- water surface ti bottom396/RConn1
  water surface ti bottom396/LConn1 -- bottom415/RConn1 -- water surface ti bottom397/RConn1
  water surface ti bottom388/RConn1 -- bottom409/RConn1 -- water surface ti bottom397/LConn1
  water surface ti bottom388/LConn1 -- bottom408/RConn1 -- water surface ti bottom389/RConn1
  water surface ti bottom389/LConn1 -- water surface ti bottom390/RConn1 -- bottom411/RConn1
  water surface ti bottom390/LConn1 -- water surface ti bottom392/RConn1 -- bottom410/RConn1
  water surface ti bottom392/LConn1 -- bottom407/RConn1 -- water surface ti bottom384/RConn1
  water surface ti bottom384/LConn1 -- water surface ti bottom387/RConn1 -- bottom404/RConn1
  water surface ti bottom386/RConn1 -- water surface ti bottom398/LConn1 -- bottom406/RConn1
  water surface ti bottom385/RConn1 -- water surface ti bottom386/LConn1 -- bottom405/RConn1
  water surface ti bottom391/RConn1 -- water surface ti bottom385/LConn1 -- bottom403/RConn1
  water surface ti bottom383/RConn1 -- water surface ti bottom391/LConn1 -- bottom402/RConn1
  water surface ti bottom383/LConn1 -- water surface ti bottom405/RConn1 -- bottom424/RConn1
  water surface ti bottom405/LConn1 -- water surface ti bottom404/RConn1 -- bottom423/RConn1
  water surface ti bottom403/RConn1 -- water surface ti bottom404/LConn1 -- bottom422/RConn1
  water surface ti bottom401/RConn1 -- water surface ti bottom403/LConn1 -- bottom421/RConn1
  water surface ti bottom400/RConn1 -- water surface ti bottom401/LConn1 -- bottom420/RConn1
  water surface ti bottom387/LConn1 -- bottom419/RConn1 -- water surface ti bottom399/RConn1
  water surface ti bottom393/RConn1 -- water surface ti bottom400/LConn1 -- bottom418/RConn1
  water surface ti bottom402/LConn1 -- water surface ti bottom382/RConn1 -- bottom400/RConn1
  Rigid Transform24/LConn1 -- bottom401/RConn1 -- Rigid Transform22/RConn1 -- water surface ti bottom393/LConn1 -- water surface ti bottom382/LConn1
  bottom412/RConn1 -- water surface ti bottom399/LConn1 -- water surface ti bottom402/RConn1
  bottom364/RConn1 -- water surface ti bottom349/RConn1
  bottom339/RConn1 -- water surface ti bottom325/RConn1
  bottom289/RConn1 -- water surface ti bottom277/RConn1
  bottom288/RConn1 -- water surface ti bottom278/RConn1
  bottom314/RConn1 -- water surface ti bottom301/RConn1
  water surface ti bottom305/RConn1 -- bottom317/RConn1
  bottom338/RConn1 -- water surface ti bottom326/RConn1
  water surface ti bottom353/RConn1 -- bottom367/RConn1
  water surface ti bottom301/LConn1 -- bottom313/RConn1 -- water surface ti bottom302/RConn1
  water surface ti bottom302/LConn1 -- water surface ti bottom303/RConn1 -- bottom316/RConn1
  water surface ti bottom303/LConn1 -- water surface ti bottom304/RConn1 -- bottom315/RConn1
  water surface ti bottom295/RConn1 -- water surface ti bottom304/LConn1 -- bottom309/RConn1
  water surface ti bottom295/LConn1 -- water surface ti bottom296/RConn1 -- bottom308/RConn1
  water surface ti bottom296/LConn1 -- bottom311/RConn1 -- water surface ti bottom297/RConn1
  water surface ti bottom297/LConn1 -- bottom310/RConn1 -- water surface ti bottom299/RConn1
  water surface ti bottom299/LConn1 -- water surface ti bottom291/RConn1 -- bottom307/RConn1
  water surface ti bottom291/LConn1 -- bottom304/RConn1 -- water surface ti bottom294/RConn1
  water surface ti bottom305/LConn1 -- water surface ti bottom293/RConn1 -- bottom306/RConn1
  water surface ti bottom293/LConn1 -- bottom305/RConn1 -- water surface ti bottom292/RConn1
  bottom303/RConn1 -- water surface ti bottom298/RConn1 -- water surface ti bottom292/LConn1
  water surface ti bottom298/LConn1 -- water surface ti bottom290/RConn1 -- bottom302/RConn1
  water surface ti bottom312/RConn1 -- water surface ti bottom290/LConn1 -- bottom324/RConn1
  water surface ti bottom311/RConn1 -- water surface ti bottom312/LConn1 -- bottom323/RConn1
  water surface ti bottom311/LConn1 -- bottom322/RConn1 -- water surface ti bottom310/RConn1
  water surface ti bottom308/RConn1 -- water surface ti bottom310/LConn1 -- bottom321/RConn1
  water surface ti bottom308/LConn1 -- bottom320/RConn1 -- water surface ti bottom307/RConn1
  water surface ti bottom294/LConn1 -- water surface ti bottom306/RConn1 -- bottom319/RConn1
  water surface ti bottom300/RConn1 -- water surface ti bottom307/LConn1 -- bottom318/RConn1
  water surface ti bottom309/LConn1 -- Rigid Transform21/RConn1 -- bottom300/RConn1 -- water surface ti bottom289/LConn1
  water surface ti bottom289/RConn1 -- water surface ti bottom300/LConn1 -- bottom301/RConn1
  water surface ti bottom306/LConn1 -- water surface ti bottom309/RConn1 -- bottom312/RConn1
  water surface ti bottom277/LConn1 -- bottom292/RConn1 -- water surface ti bottom281/RConn1
  water surface ti bottom278/LConn1 -- water surface ti bottom279/RConn1 -- bottom291/RConn1
  water surface ti bottom279/LConn1 -- water surface ti bottom280/RConn1 -- bottom290/RConn1
  water surface ti bottom271/RConn1 -- water surface ti bottom280/LConn1 -- bottom284/RConn1
  water surface ti bottom271/LConn1 -- water surface ti bottom272/RConn1 -- bottom283/RConn1
  water surface ti bottom272/LConn1 -- bottom286/RConn1 -- water surface ti bottom273/RConn1
  water surface ti bottom273/LConn1 -- bottom285/RConn1 -- water surface ti bottom275/RConn1
  water surface ti bottom275/LConn1 -- water surface ti bottom267/RConn1 -- bottom282/RConn1
  water surface ti bottom267/LConn1 -- bottom279/RConn1 -- water surface ti bottom270/RConn1
  water surface ti bottom269/RConn1 -- bottom281/RConn1 -- water surface ti bottom281/LConn1
  water surface ti bottom268/RConn1 -- bottom280/RConn1 -- water surface ti bottom269/LConn1
  water surface ti bottom274/RConn1 -- bottom278/RConn1 -- water surface ti bottom268/LConn1
  water surface ti bottom266/RConn1 -- bottom277/RConn1 -- water surface ti bottom274/LConn1
  water surface ti bottom266/LConn1 -- bottom299/RConn1 -- water surface ti bottom288/RConn1
  water surface ti bottom288/LConn1 -- bottom298/RConn1 -- water surface ti bottom287/RConn1
  water surface ti bottom286/RConn1 -- bottom297/RConn1 -- water surface ti bottom287/LConn1
  water surface ti bottom284/RConn1 -- bottom296/RConn1 -- water surface ti bottom286/LConn1
  water surface ti bottom283/RConn1 -- bottom295/RConn1 -- water surface ti bottom284/LConn1
  water surface ti bottom270/LConn1 -- water surface ti bottom282/RConn1 -- bottom294/RConn1
  water surface ti bottom276/RConn1 -- bottom293/RConn1 -- water surface ti bottom283/LConn1
  water surface ti bottom285/LConn1 -- bottom275/RConn1 -- water surface ti bottom265/RConn1
  Rigid Transform21/LConn1 -- Rigid Transform19/RConn1 -- bottom276/RConn1 -- water surface ti bottom265/LConn1 -- water surface ti bottom276/LConn1
  bottom287/RConn1 -- water surface ti bottom285/RConn1 -- water surface ti bottom282/LConn1
  water surface ti bottom349/LConn1 -- water surface ti bottom350/RConn1 -- bottom363/RConn1
  water surface ti bottom350/LConn1 -- bottom366/RConn1 -- water surface ti bottom351/RConn1
  water surface ti bottom351/LConn1 -- bottom365/RConn1 -- water surface ti bottom352/RConn1
  water surface ti bottom343/RConn1 -- bottom359/RConn1 -- water surface ti bottom352/LConn1
  water surface ti bottom343/LConn1 -- bottom358/RConn1 -- water surface ti bottom344/RConn1
  water surface ti bottom344/LConn1 -- water surface ti bottom345/RConn1 -- bottom361/RConn1
  water surface ti bottom345/LConn1 -- water surface ti bottom347/RConn1 -- bottom360/RConn1
  water surface ti bottom347/LConn1 -- bottom357/RConn1 -- water surface ti bottom339/RConn1
  water surface ti bottom339/LConn1 -- water surface ti bottom342/RConn1 -- bottom354/RConn1
  water surface ti bottom353/LConn1 -- bottom356/RConn1 -- water surface ti bottom341/RConn1
  water surface ti bottom341/LConn1 -- water surface ti bottom340/RConn1 -- bottom355/RConn1
  bottom353/RConn1 -- water surface ti bottom340/LConn1 -- water surface ti bottom346/RConn1
  water surface ti bottom346/LConn1 -- bottom352/RConn1 -- water surface ti bottom338/RConn1
  water surface ti bottom360/RConn1 -- bottom374/RConn1 -- water surface ti bottom338/LConn1
  water surface ti bottom359/RConn1 -- bottom373/RConn1 -- water surface ti bottom360/LConn1
  water surface ti bottom359/LConn1 -- water surface ti bottom358/RConn1 -- bottom372/RConn1
  water surface ti bottom356/RConn1 -- bottom371/RConn1 -- water surface ti bottom358/LConn1
  water surface ti bottom356/LConn1 -- water surface ti bottom355/RConn1 -- bottom370/RConn1
  water surface ti bottom342/LConn1 -- bottom369/RConn1 -- water surface ti bottom354/RConn1
  water surface ti bottom348/RConn1 -- bottom368/RConn1 -- water surface ti bottom355/LConn1
  water surface ti bottom337/LConn1 -- water surface ti bottom357/LConn1 -- bottom350/RConn1 -- Rigid Transform18/RConn1 -- Rigid Transform19/LConn1
  water surface ti bottom337/RConn1 -- bottom351/RConn1 -- water surface ti bottom348/LConn1
  water surface ti bottom354/LConn1 -- bottom362/RConn1 -- water surface ti bottom357/RConn1
  water surface ti bottom325/LConn1 -- water surface ti bottom329/RConn1 -- bottom342/RConn1
  water surface ti bottom326/LConn1 -- bottom341/RConn1 -- water surface ti bottom327/RConn1
  water surface ti bottom327/LConn1 -- bottom340/RConn1 -- water surface ti bottom328/RConn1
  water surface ti bottom319/RConn1 -- bottom334/RConn1 -- water surface ti bottom328/LConn1
  water surface ti bottom319/LConn1 -- bottom333/RConn1 -- water surface ti bottom320/RConn1
  water surface ti bottom320/LConn1 -- water surface ti bottom321/RConn1 -- bottom336/RConn1
  water surface ti bottom321/LConn1 -- water surface ti bottom323/RConn1 -- bottom335/RConn1
  water surface ti bottom323/LConn1 -- bottom332/RConn1 -- water surface ti bottom315/RConn1
  water surface ti bottom315/LConn1 -- water surface ti bottom318/RConn1 -- bottom329/RConn1
  water surface ti bottom317/RConn1 -- water surface ti bottom329/LConn1 -- bottom331/RConn1
  water surface ti bottom316/RConn1 -- water surface ti bottom317/LConn1 -- bottom330/RConn1
  water surface ti bottom322/RConn1 -- water surface ti bottom316/LConn1 -- bottom328/RConn1
  water surface ti bottom314/RConn1 -- water surface ti bottom322/LConn1 -- bottom327/RConn1
  water surface ti bottom314/LConn1 -- water surface ti bottom336/RConn1 -- bottom349/RConn1
  water surface ti bottom336/LConn1 -- water surface ti bottom335/RConn1 -- bottom348/RConn1
  water surface ti bottom334/RConn1 -- water surface ti bottom335/LConn1 -- bottom347/RConn1
  water surface ti bottom332/RConn1 -- water surface ti bottom334/LConn1 -- bottom346/RConn1
  water surface ti bottom331/RConn1 -- water surface ti bottom332/LConn1 -- bottom345/RConn1
  water surface ti bottom318/LConn1 -- bottom344/RConn1 -- water surface ti bottom330/RConn1
  water surface ti bottom324/RConn1 -- water surface ti bottom331/LConn1 -- bottom343/RConn1
  water surface ti bottom333/LConn1 -- water surface ti bottom313/RConn1 -- bottom325/RConn1
  Rigid Transform18/LConn1 -- water surface ti bottom313/LConn1 -- bottom326/RConn1 -- Rigid Transform16/RConn1 -- water surface ti bottom324/LConn1
  bottom337/RConn1 -- water surface ti bottom330/LConn1 -- water surface ti bottom333/RConn1
  bottom239/RConn1 -- water surface ti bottom229/RConn1
  bottom238/RConn1 -- water surface ti bottom230/RConn1
  bottom264/RConn1 -- water surface ti bottom253/RConn1
  water surface ti bottom257/RConn1 -- bottom267/RConn1
  water surface ti bottom209/RConn1 -- bottom217/RConn1
  bottom214/RConn1 -- water surface ti bottom205/RConn1
  bottom188/RConn1 -- water surface ti bottom182/RConn1
  bottom189/RConn1 -- water surface ti bottom181/RConn1
  water surface ti bottom205/LConn1 -- water surface ti bottom206/RConn1 -- bottom213/RConn1
  water surface ti bottom206/LConn1 -- bottom216/RConn1 -- water surface ti bottom207/RConn1
  water surface ti bottom207/LConn1 -- bottom215/RConn1 -- water surface ti bottom208/RConn1
  water surface ti bottom199/RConn1 -- bottom209/RConn1 -- water surface ti bottom208/LConn1
  water surface ti bottom199/LConn1 -- bottom208/RConn1 -- water surface ti bottom200/RConn1
  water surface ti bottom200/LConn1 -- water surface ti bottom201/RConn1 -- bottom211/RConn1
  water surface ti bottom201/LConn1 -- water surface ti bottom203/RConn1 -- bottom210/RConn1
  water surface ti bottom203/LConn1 -- bottom207/RConn1 -- water surface ti bottom195/RConn1
  water surface ti bottom195/LConn1 -- water surface ti bottom198/RConn1 -- bottom204/RConn1
  water surface ti bottom209/LConn1 -- bottom206/RConn1 -- water surface ti bottom197/RConn1
  water surface ti bottom197/LConn1 -- water surface ti bottom196/RConn1 -- bottom205/RConn1
  bottom203/RConn1 -- water surface ti bottom196/LConn1 -- water surface ti bottom202/RConn1
  water surface ti bottom202/LConn1 -- bottom202/RConn1 -- water surface ti bottom194/RConn1
  water surface ti bottom216/RConn1 -- bottom224/RConn1 -- water surface ti bottom194/LConn1
  water surface ti bottom215/RConn1 -- bottom223/RConn1 -- water surface ti bottom216/LConn1
  water surface ti bottom215/LConn1 -- water surface ti bottom214/RConn1 -- bottom222/RConn1
  water surface ti bottom212/RConn1 -- bottom221/RConn1 -- water surface ti bottom214/LConn1
  water surface ti bottom212/LConn1 -- water surface ti bottom211/RConn1 -- bottom220/RConn1
  water surface ti bottom198/LConn1 -- bottom219/RConn1 -- water surface ti bottom210/RConn1
  water surface ti bottom204/RConn1 -- bottom218/RConn1 -- water surface ti bottom211/LConn1
  Rigid Transform15/RConn1 -- water surface ti bottom213/LConn1 -- Rigid Transform16/LConn1 -- water surface ti bottom193/LConn1 -- bottom200/RConn1
  water surface ti bottom193/RConn1 -- bottom201/RConn1 -- water surface ti bottom204/LConn1
  water surface ti bottom210/LConn1 -- bottom212/RConn1 -- water surface ti bottom213/RConn1
  water surface ti bottom181/LConn1 -- water surface ti bottom185/RConn1 -- bottom192/RConn1
  water surface ti bottom182/LConn1 -- bottom191/RConn1 -- water surface ti bottom183/RConn1
  water surface ti bottom183/LConn1 -- bottom190/RConn1 -- water surface ti bottom184/RConn1
  water surface ti bottom175/RConn1 -- bottom184/RConn1 -- water surface ti bottom184/LConn1
  water surface ti bottom175/LConn1 -- bottom183/RConn1 -- water surface ti bottom176/RConn1
  water surface ti bottom176/LConn1 -- water surface ti bottom177/RConn1 -- bottom186/RConn1
  water surface ti bottom177/LConn1 -- water surface ti bottom179/RConn1 -- bottom185/RConn1
  water surface ti bottom179/LConn1 -- bottom182/RConn1 -- water surface ti bottom171/RConn1
  water surface ti bottom171/LConn1 -- water surface ti bottom174/RConn1 -- bottom179/RConn1
  water surface ti bottom173/RConn1 -- water surface ti bottom185/LConn1 -- bottom181/RConn1
  water surface ti bottom172/RConn1 -- water surface ti bottom173/LConn1 -- bottom180/RConn1
  water surface ti bottom178/RConn1 -- water surface ti bottom172/LConn1 -- bottom178/RConn1
  water surface ti bottom170/RConn1 -- water surface ti bottom178/LConn1 -- bottom177/RConn1
  water surface ti bottom170/LConn1 -- water surface ti bottom192/RConn1 -- bottom199/RConn1
  water surface ti bottom192/LConn1 -- water surface ti bottom191/RConn1 -- bottom198/RConn1
  water surface ti bottom190/RConn1 -- water surface ti bottom191/LConn1 -- bottom197/RConn1
  water surface ti bottom188/RConn1 -- water surface ti bottom190/LConn1 -- bottom196/RConn1
  water surface ti bottom187/RConn1 -- water surface ti bottom188/LConn1 -- bottom195/RConn1
  water surface ti bottom174/LConn1 -- bottom194/RConn1 -- water surface ti bottom186/RConn1
  water surface ti bottom180/RConn1 -- water surface ti bottom187/LConn1 -- bottom193/RConn1
  water surface ti bottom189/LConn1 -- water surface ti bottom169/RConn1 -- bottom175/RConn1
  water surface ti bottom169/LConn1 -- bottom176/RConn1 -- Rigid Transform13/RConn1 -- water surface ti bottom180/LConn1 -- Rigid Transform15/LConn1
  bottom187/RConn1 -- water surface ti bottom186/LConn1 -- water surface ti bottom189/RConn1
  water surface ti bottom253/LConn1 -- bottom263/RConn1 -- water surface ti bottom254/RConn1
  water surface ti bottom254/LConn1 -- water surface ti bottom255/RConn1 -- bottom266/RConn1
  water surface ti bottom255/LConn1 -- water surface ti bottom256/RConn1 -- bottom265/RConn1
  water surface ti bottom247/RConn1 -- water surface ti bottom256/LConn1 -- bottom259/RConn1
  water surface ti bottom247/LConn1 -- water surface ti bottom248/RConn1 -- bottom258/RConn1
  water surface ti bottom248/LConn1 -- bottom261/RConn1 -- water surface ti bottom249/RConn1
  water surface ti bottom249/LConn1 -- bottom260/RConn1 -- water surface ti bottom251/RConn1
  water surface ti bottom251/LConn1 -- water surface ti bottom243/RConn1 -- bottom257/RConn1
  water surface ti bottom243/LConn1 -- bottom254/RConn1 -- water surface ti bottom246/RConn1
  water surface ti bottom257/LConn1 -- water surface ti bottom245/RConn1 -- bottom256/RConn1
  water surface ti bottom245/LConn1 -- bottom255/RConn1 -- water surface ti bottom244/RConn1
  bottom253/RConn1 -- water surface ti bottom250/RConn1 -- water surface ti bottom244/LConn1
  water surface ti bottom250/LConn1 -- water surface ti bottom242/RConn1 -- bottom252/RConn1
  water surface ti bottom264/RConn1 -- water surface ti bottom242/LConn1 -- bottom274/RConn1
  water surface ti bottom263/RConn1 -- water surface ti bottom264/LConn1 -- bottom273/RConn1
  water surface ti bottom263/LConn1 -- bottom272/RConn1 -- water surface ti bottom262/RConn1
  water surface ti bottom260/RConn1 -- water surface ti bottom262/LConn1 -- bottom271/RConn1
  water surface ti bottom260/LConn1 -- bottom270/RConn1 -- water surface ti bottom259/RConn1
  water surface ti bottom246/LConn1 -- water surface ti bottom258/RConn1 -- bottom269/RConn1
  water surface ti bottom252/RConn1 -- water surface ti bottom259/LConn1 -- bottom268/RConn1
  bottom250/RConn1 -- water surface ti bottom261/LConn1 -- water surface ti bottom241/LConn1 -- Rigid Transform13/LConn1 -- Rigid Transform12/RConn1
  water surface ti bottom241/RConn1 -- water surface ti bottom252/LConn1 -- bottom251/RConn1
  water surface ti bottom258/LConn1 -- water surface ti bottom261/RConn1 -- bottom262/RConn1
  water surface ti bottom229/LConn1 -- bottom242/RConn1 -- water surface ti bottom233/RConn1
  water surface ti bottom230/LConn1 -- water surface ti bottom231/RConn1 -- bottom241/RConn1
  water surface ti bottom231/LConn1 -- water surface ti bottom232/RConn1 -- bottom240/RConn1
  water surface ti bottom223/RConn1 -- water surface ti bottom232/LConn1 -- bottom234/RConn1
  water surface ti bottom223/LConn1 -- water surface ti bottom224/RConn1 -- bottom233/RConn1
  water surface ti bottom224/LConn1 -- bottom236/RConn1 -- water surface ti bottom225/RConn1
  water surface ti bottom225/LConn1 -- bottom235/RConn1 -- water surface ti bottom227/RConn1
  water surface ti bottom227/LConn1 -- water surface ti bottom219/RConn1 -- bottom232/RConn1
  water surface ti bottom219/LConn1 -- bottom229/RConn1 -- water surface ti bottom222/RConn1
  water surface ti bottom221/RConn1 -- bottom231/RConn1 -- water surface ti bottom233/LConn1
  water surface ti bottom220/RConn1 -- bottom230/RConn1 -- water surface ti bottom221/LConn1
  water surface ti bottom226/RConn1 -- bottom228/RConn1 -- water surface ti bottom220/LConn1
  water surface ti bottom218/RConn1 -- bottom227/RConn1 -- water surface ti bottom226/LConn1
  water surface ti bottom218/LConn1 -- bottom249/RConn1 -- water surface ti bottom240/RConn1
  water surface ti bottom240/LConn1 -- bottom248/RConn1 -- water surface ti bottom239/RConn1
  water surface ti bottom238/RConn1 -- bottom247/RConn1 -- water surface ti bottom239/LConn1
  water surface ti bottom236/RConn1 -- bottom246/RConn1 -- water surface ti bottom238/LConn1
  water surface ti bottom235/RConn1 -- bottom245/RConn1 -- water surface ti bottom236/LConn1
  water surface ti bottom222/LConn1 -- water surface ti bottom234/RConn1 -- bottom244/RConn1
  water surface ti bottom228/RConn1 -- bottom243/RConn1 -- water surface ti bottom235/LConn1
  water surface ti bottom237/LConn1 -- bottom225/RConn1 -- water surface ti bottom217/RConn1
  Rigid Transform12/LConn1 -- water surface ti bottom228/LConn1 -- water surface ti bottom217/LConn1 -- bottom226/RConn1 -- Rigid Transform10/RConn1
  bottom237/RConn1 -- water surface ti bottom237/RConn1 -- water surface ti bottom234/LConn1
  bottom139/RConn1 -- water surface ti bottom133/RConn1
  bottom138/RConn1 -- water surface ti bottom134/RConn1
  bottom164/RConn1 -- water surface ti bottom157/RConn1
  water surface ti bottom161/RConn1 -- bottom167/RConn1
  water surface ti bottom157/LConn1 -- bottom163/RConn1 -- water surface ti bottom158/RConn1
  water surface ti bottom158/LConn1 -- water surface ti bottom159/RConn1 -- bottom166/RConn1
  water surface ti bottom159/LConn1 -- water surface ti bottom160/RConn1 -- bottom165/RConn1
  water surface ti bottom151/RConn1 -- water surface ti bottom160/LConn1 -- bottom159/RConn1
  water surface ti bottom151/LConn1 -- water surface ti bottom152/RConn1 -- bottom158/RConn1
  water surface ti bottom152/LConn1 -- bottom161/RConn1 -- water surface ti bottom153/RConn1
  water surface ti bottom153/LConn1 -- bottom160/RConn1 -- water surface ti bottom155/RConn1
  water surface ti bottom155/LConn1 -- water surface ti bottom147/RConn1 -- bottom157/RConn1
  water surface ti bottom147/LConn1 -- bottom154/RConn1 -- water surface ti bottom150/RConn1
  water surface ti bottom161/LConn1 -- water surface ti bottom149/RConn1 -- bottom156/RConn1
  water surface ti bottom149/LConn1 -- bottom155/RConn1 -- water surface ti bottom148/RConn1
  bottom153/RConn1 -- water surface ti bottom154/RConn1 -- water surface ti bottom148/LConn1
  water surface ti bottom154/LConn1 -- water surface ti bottom146/RConn1 -- bottom152/RConn1
  water surface ti bottom168/RConn1 -- water surface ti bottom146/LConn1 -- bottom174/RConn1
  water surface ti bottom167/RConn1 -- water surface ti bottom168/LConn1 -- bottom173/RConn1
  water surface ti bottom167/LConn1 -- bottom172/RConn1 -- water surface ti bottom166/RConn1
  water surface ti bottom164/RConn1 -- water surface ti bottom166/LConn1 -- bottom171/RConn1
  water surface ti bottom164/LConn1 -- bottom170/RConn1 -- water surface ti bottom163/RConn1
  water surface ti bottom150/LConn1 -- water surface ti bottom162/RConn1 -- bottom169/RConn1
  water surface ti bottom156/RConn1 -- water surface ti bottom163/LConn1 -- bottom168/RConn1
  Rigid Transform9/RConn1 -- bottom150/RConn1 -- water surface ti bottom165/LConn1 -- Rigid Transform10/LConn1 -- water surface ti bottom145/LConn1
  water surface ti bottom145/RConn1 -- water surface ti bottom156/LConn1 -- bottom151/RConn1
  water surface ti bottom162/LConn1 -- water surface ti bottom165/RConn1 -- bottom162/RConn1
  water surface ti bottom133/LConn1 -- bottom142/RConn1 -- water surface ti bottom137/RConn1
  water surface ti bottom134/LConn1 -- water surface ti bottom135/RConn1 -- bottom141/RConn1
  water surface ti bottom135/LConn1 -- water surface ti bottom136/RConn1 -- bottom140/RConn1
  water surface ti bottom127/RConn1 -- water surface ti bottom136/LConn1 -- bottom134/RConn1
  water surface ti bottom127/LConn1 -- water surface ti bottom128/RConn1 -- bottom133/RConn1
  water surface ti bottom128/LConn1 -- bottom136/RConn1 -- water surface ti bottom129/RConn1
  water surface ti bottom129/LConn1 -- bottom135/RConn1 -- water surface ti bottom131/RConn1
  water surface ti bottom131/LConn1 -- water surface ti bottom123/RConn1 -- bottom132/RConn1
  water surface ti bottom123/LConn1 -- bottom129/RConn1 -- water surface ti bottom126/RConn1
  water surface ti bottom125/RConn1 -- bottom131/RConn1 -- water surface ti bottom137/LConn1
  water surface ti bottom124/RConn1 -- bottom130/RConn1 -- water surface ti bottom125/LConn1
  water surface ti bottom130/RConn1 -- bottom128/RConn1 -- water surface ti bottom124/LConn1
  water surface ti bottom122/RConn1 -- bottom127/RConn1 -- water surface ti bottom130/LConn1
  water surface ti bottom122/LConn1 -- bottom149/RConn1 -- water surface ti bottom144/RConn1
  water surface ti bottom144/LConn1 -- bottom148/RConn1 -- water surface ti bottom143/RConn1
  water surface ti bottom142/RConn1 -- bottom147/RConn1 -- water surface ti bottom143/LConn1
  water surface ti bottom140/RConn1 -- bottom146/RConn1 -- water surface ti bottom142/LConn1
  water surface ti bottom139/RConn1 -- bottom145/RConn1 -- water surface ti bottom140/LConn1
  water surface ti bottom126/LConn1 -- water surface ti bottom138/RConn1 -- bottom144/RConn1
  water surface ti bottom132/RConn1 -- bottom143/RConn1 -- water surface ti bottom139/LConn1
  water surface ti bottom141/LConn1 -- bottom125/RConn1 -- water surface ti bottom121/RConn1
  water surface ti bottom121/LConn1 -- water surface ti bottom132/LConn1 -- Rigid Transform9/LConn1 -- bottom126/RConn1 -- Rigid Transform7/RConn1
  bottom137/RConn1 -- water surface ti bottom141/RConn1 -- water surface ti bottom138/LConn1
  bottom114/RConn1 -- water surface ti bottom109/RConn1
  water surface ti bottom113/RConn1 -- bottom117/RConn1
  water surface ti bottom109/LConn1 -- bottom113/RConn1 -- water surface ti bottom110/RConn1
  water surface ti bottom110/LConn1 -- water surface ti bottom111/RConn1 -- bottom116/RConn1
  water surface ti bottom111/LConn1 -- water surface ti bottom112/RConn1 -- bottom115/RConn1
  water surface ti bottom103/RConn1 -- water surface ti bottom112/LConn1 -- bottom109/RConn1
  water surface ti bottom103/LConn1 -- water surface ti bottom104/RConn1 -- bottom108/RConn1
  water surface ti bottom104/LConn1 -- bottom111/RConn1 -- water surface ti bottom105/RConn1
  water surface ti bottom105/LConn1 -- bottom110/RConn1 -- water surface ti bottom107/RConn1
  water surface ti bottom107/LConn1 -- water surface ti bottom99/RConn1 -- bottom107/RConn1
  water surface ti bottom99/LConn1 -- bottom104/RConn1 -- water surface ti bottom102/RConn1
  water surface ti bottom113/LConn1 -- water surface ti bottom101/RConn1 -- bottom106/RConn1
  water surface ti bottom101/LConn1 -- bottom105/RConn1 -- water surface ti bottom100/RConn1
  bottom103/RConn1 -- water surface ti bottom106/RConn1 -- water surface ti bottom100/LConn1
  water surface ti bottom106/LConn1 -- water surface ti bottom98/RConn1 -- bottom102/RConn1
  water surface ti bottom120/RConn1 -- water surface ti bottom98/LConn1 -- bottom124/RConn1
  water surface ti bottom119/RConn1 -- water surface ti bottom120/LConn1 -- bottom123/RConn1
  water surface ti bottom119/LConn1 -- bottom122/RConn1 -- water surface ti bottom118/RConn1
  water surface ti bottom116/RConn1 -- water surface ti bottom118/LConn1 -- bottom121/RConn1
  water surface ti bottom116/LConn1 -- bottom120/RConn1 -- water surface ti bottom115/RConn1
  water surface ti bottom102/LConn1 -- water surface ti bottom114/RConn1 -- bottom119/RConn1
  water surface ti bottom108/RConn1 -- water surface ti bottom115/LConn1 -- bottom118/RConn1
  Rigid Transform22/LConn1 -- bottom100/RConn1 -- water surface ti bottom117/LConn1 -- Rigid Transform6/RConn1 -- water surface ti bottom97/LConn1
  water surface ti bottom97/RConn1 -- water surface ti bottom108/LConn1 -- bottom101/RConn1
  water surface ti bottom114/LConn1 -- water surface ti bottom117/RConn1 -- bottom112/RConn1
  water surface ti bottom89/RConn1 -- bottom92/RConn1
  bottom89/RConn1 -- water surface ti bottom85/RConn1
  water surface ti bottom85/LConn1 -- water surface ti bottom86/RConn1 -- bottom88/RConn1
  water surface ti bottom86/LConn1 -- bottom91/RConn1 -- water surface ti bottom87/RConn1
  water surface ti bottom87/LConn1 -- bottom90/RConn1 -- water surface ti bottom88/RConn1
  water surface ti bottom79/RConn1 -- bottom84/RConn1 -- water surface ti bottom88/LConn1
  water surface ti bottom79/LConn1 -- bottom83/RConn1 -- water surface ti bottom80/RConn1
  water surface ti bottom80/LConn1 -- water surface ti bottom81/RConn1 -- bottom86/RConn1
  water surface ti bottom81/LConn1 -- water surface ti bottom83/RConn1 -- bottom85/RConn1
  water surface ti bottom83/LConn1 -- bottom82/RConn1 -- water surface ti bottom75/RConn1
  water surface ti bottom75/LConn1 -- water surface ti bottom78/RConn1 -- bottom79/RConn1
  water surface ti bottom89/LConn1 -- bottom81/RConn1 -- water surface ti bottom77/RConn1
  water surface ti bottom77/LConn1 -- water surface ti bottom76/RConn1 -- bottom80/RConn1
  bottom78/RConn1 -- water surface ti bottom76/LConn1 -- water surface ti bottom82/RConn1
  water surface ti bottom82/LConn1 -- bottom77/RConn1 -- water surface ti bottom74/RConn1
  water surface ti bottom96/RConn1 -- bottom99/RConn1 -- water surface ti bottom74/LConn1
  water surface ti bottom95/RConn1 -- bottom98/RConn1 -- water surface ti bottom96/LConn1
  water surface ti bottom95/LConn1 -- water surface ti bottom94/RConn1 -- bottom97/RConn1
  water surface ti bottom92/RConn1 -- bottom96/RConn1 -- water surface ti bottom94/LConn1
  water surface ti bottom92/LConn1 -- water surface ti bottom91/RConn1 -- bottom95/RConn1
  water surface ti bottom78/LConn1 -- bottom94/RConn1 -- water surface ti bottom90/RConn1
  water surface ti bottom84/RConn1 -- bottom93/RConn1 -- water surface ti bottom91/LConn1
  water surface ti bottom93/LConn1 -- bottom75/RConn1 -- Rigid Transform5/RConn1 -- Rigid Transform7/LConn1 -- water surface ti bottom73/LConn1
  water surface ti bottom73/RConn1 -- bottom76/RConn1 -- water surface ti bottom84/LConn1
  water surface ti bottom90/LConn1 -- bottom87/RConn1 -- water surface ti bottom93/RConn1
  bottom64/RConn1 -- water surface ti bottom61/RConn1
  bottom63/RConn1 -- water surface ti bottom62/RConn1
  water surface ti bottom61/LConn1 -- bottom67/RConn1 -- water surface ti bottom65/RConn1
  water surface ti bottom62/LConn1 -- water surface ti bottom63/RConn1 -- bottom66/RConn1
  water surface ti bottom63/LConn1 -- water surface ti bottom64/RConn1 -- bottom65/RConn1
  water surface ti bottom55/RConn1 -- water surface ti bottom64/LConn1 -- bottom59/RConn1
  water surface ti bottom55/LConn1 -- water surface ti bottom56/RConn1 -- bottom58/RConn1
  water surface ti bottom56/LConn1 -- bottom61/RConn1 -- water surface ti bottom57/RConn1
  water surface ti bottom57/LConn1 -- bottom60/RConn1 -- water surface ti bottom59/RConn1
  water surface ti bottom59/LConn1 -- water surface ti bottom51/RConn1 -- bottom57/RConn1
  water surface ti bottom51/LConn1 -- bottom54/RConn1 -- water surface ti bottom54/RConn1
  water surface ti bottom53/RConn1 -- bottom56/RConn1 -- water surface ti bottom65/LConn1
  water surface ti bottom52/RConn1 -- bottom55/RConn1 -- water surface ti bottom53/LConn1
  water surface ti bottom58/RConn1 -- bottom53/RConn1 -- water surface ti bottom52/LConn1
  water surface ti bottom50/RConn1 -- bottom52/RConn1 -- water surface ti bottom58/LConn1
  water surface ti bottom50/LConn1 -- bottom74/RConn1 -- water surface ti bottom72/RConn1
  water surface ti bottom72/LConn1 -- bottom73/RConn1 -- water surface ti bottom71/RConn1
  water surface ti bottom70/RConn1 -- bottom72/RConn1 -- water surface ti bottom71/LConn1
  water surface ti bottom68/RConn1 -- bottom71/RConn1 -- water surface ti bottom70/LConn1
  water surface ti bottom67/RConn1 -- bottom70/RConn1 -- water surface ti bottom68/LConn1
  water surface ti bottom54/LConn1 -- water surface ti bottom66/RConn1 -- bottom69/RConn1
  water surface ti bottom60/RConn1 -- bottom68/RConn1 -- water surface ti bottom67/LConn1
  water surface ti bottom69/LConn1 -- bottom50/RConn1 -- water surface ti bottom49/RConn1
  water surface ti bottom60/LConn1 -- bottom51/RConn1 -- Rigid Transform6/LConn1 -- water surface ti bottom49/LConn1 -- Rigid Transform2/RConn1
  bottom62/RConn1 -- water surface ti bottom69/RConn1 -- water surface ti bottom66/LConn1
  bottom39/RConn1 -- water surface ti bottom37/RConn1
  bottom42/RConn1 -- water surface ti bottom37/LConn1 -- water surface ti bottom41/RConn1
  bottom38/RConn1 -- water surface ti bottom38/RConn1
  water surface ti bottom38/LConn1 -- bottom41/RConn1 -- water surface ti bottom39/RConn1
  water surface ti bottom39/LConn1 -- bottom40/RConn1 -- water surface ti bottom40/RConn1
  water surface ti bottom31/RConn1 -- bottom34/RConn1 -- water surface ti bottom40/LConn1
  water surface ti bottom31/LConn1 -- bottom33/RConn1 -- water surface ti bottom32/RConn1
  water surface ti bottom32/LConn1 -- water surface ti bottom33/RConn1 -- bottom36/RConn1
  water surface ti bottom33/LConn1 -- water surface ti bottom35/RConn1 -- bottom35/RConn1
  water surface ti bottom35/LConn1 -- bottom32/RConn1 -- water surface ti bottom27/RConn1
  water surface ti bottom27/LConn1 -- water surface ti bottom30/RConn1 -- bottom29/RConn1
  bottom31/RConn1 -- water surface ti bottom41/LConn1 -- water surface ti bottom29/RConn1
  water surface ti bottom28/RConn1 -- water surface ti bottom29/LConn1 -- bottom30/RConn1
  bottom28/RConn1 -- water surface ti bottom28/LConn1 -- water surface ti bottom34/RConn1
  bottom27/RConn1 -- water surface ti bottom34/LConn1 -- water surface ti bottom26/RConn1
  bottom49/RConn1 -- water surface ti bottom48/RConn1 -- water surface ti bottom26/LConn1
  bottom48/RConn1 -- water surface ti bottom47/RConn1 -- water surface ti bottom48/LConn1
  water surface ti bottom46/RConn1 -- water surface ti bottom47/LConn1 -- bottom47/RConn1
  bottom46/RConn1 -- water surface ti bottom44/RConn1 -- water surface ti bottom46/LConn1
  water surface ti bottom43/RConn1 -- water surface ti bottom44/LConn1 -- bottom45/RConn1
  water surface ti bottom30/LConn1 -- bottom44/RConn1 -- water surface ti bottom42/RConn1
  bottom43/RConn1 -- water surface ti bottom36/RConn1 -- water surface ti bottom43/LConn1
  bottom25/RConn1 -- water surface ti bottom25/RConn1 -- water surface ti bottom45/LConn1
  Rigid Transform5/LConn1 -- bottom26/RConn1 -- Rigid Transform1/RConn1 -- water surface ti bottom25/LConn1 -- water surface ti bottom36/LConn1
  bottom37/RConn1 -- water surface ti bottom42/LConn1 -- water surface ti bottom45/RConn1
  water surface ti bottom24/RConn1 -- bottom24/RConn1
  bottom21/RConn1 -- water surface ti bottom20/RConn1
  water surface ti bottom20/LConn1 -- bottom20/RConn1 -- water surface ti bottom21/RConn1
  water surface ti bottom21/LConn1 -- water surface ti bottom22/RConn1 -- bottom23/RConn1
  water surface ti bottom22/LConn1 -- water surface ti bottom23/RConn1 -- bottom22/RConn1
  water surface ti bottom15/RConn1 -- water surface ti bottom23/LConn1 -- bottom17/RConn1
  water surface ti bottom15/LConn1 -- water surface ti bottom16/RConn1 -- bottom16/RConn1
  water surface ti bottom16/LConn1 -- bottom19/RConn1 -- water surface ti bottom17/RConn1
  water surface ti bottom17/LConn1 -- bottom18/RConn1 -- water surface ti bottom19/RConn1
  water surface ti bottom19/LConn1 -- water surface ti bottom11/RConn1 -- bottom15/RConn1
  water surface ti bottom11/LConn1 -- bottom12/RConn1 -- water surface ti bottom14/RConn1
  bottom14/RConn1 -- water surface ti bottom24/LConn1 -- water surface ti bottom13/RConn1
  water surface ti bottom13/LConn1 -- bottom13/RConn1 -- water surface ti bottom12/RConn1
  bottom11/RConn1 -- water surface ti bottom18/RConn1 -- water surface ti bottom12/LConn1
  bottom10/RConn1 -- water surface ti bottom18/LConn1 -- water surface ti bottom10/RConn1
  water surface ti bottom9/RConn1 -- water surface ti bottom10/LConn1 -- bottom9/RConn1
  bottom8/RConn1 -- water surface ti bottom9/LConn1 -- water surface ti bottom8/RConn1
  water surface ti bottom8/LConn1 -- bottom7/RConn1 -- water surface ti bottom7/RConn1
  bottom6/RConn1 -- water surface ti bottom7/LConn1 -- water surface ti bottom5/RConn1
  water surface ti bottom5/LConn1 -- bottom5/RConn1 -- water surface ti bottom4/RConn1
  water surface ti bottom14/LConn1 -- water surface ti bottom3/RConn1 -- bottom4/RConn1
  bottom3/RConn1 -- water surface ti bottom4/LConn1 -- water surface ti bottom2/RConn1
  Brick Solid/RConn1 -- bottom/RConn1 -- Rigid Transform/RConn1 -- Rigid Transform2/LConn1 -- water surface ti bottom1/LConn1 -- Rigid Transform1/LConn1 -- water surface ti bottom6/LConn1
  bottom1/RConn1 -- water surface ti bottom2/LConn1 -- water surface ti bottom1/RConn1
  water surface ti bottom3/LConn1 -- water surface ti bottom6/RConn1 -- bottom2/RConn1
  From World/RConn1 -- Rigid Transform/LConn1
